simulink model "testingMotorModel"  (R2020b)
settings: Solver=VariableStepAuto  StartTime=0.0  StopTime=10  RelTol=1e-3
values from neighbouring files (symbols this model uses):
  A = motorSS.A    [doingActualControlTheory.m]
  B = motorSS.B    [doingActualControlTheory.m]
  C = motorSS.C    [doingActualControlTheory.m]
  D = motorSS.D    [doingActualControlTheory.m]
  Kr = K(1)    [doingActualControlTheory.m]
  Kx = K(2)    [doingActualControlTheory.m]
settings Model: Creator=drago  LastModifiedBy=drago

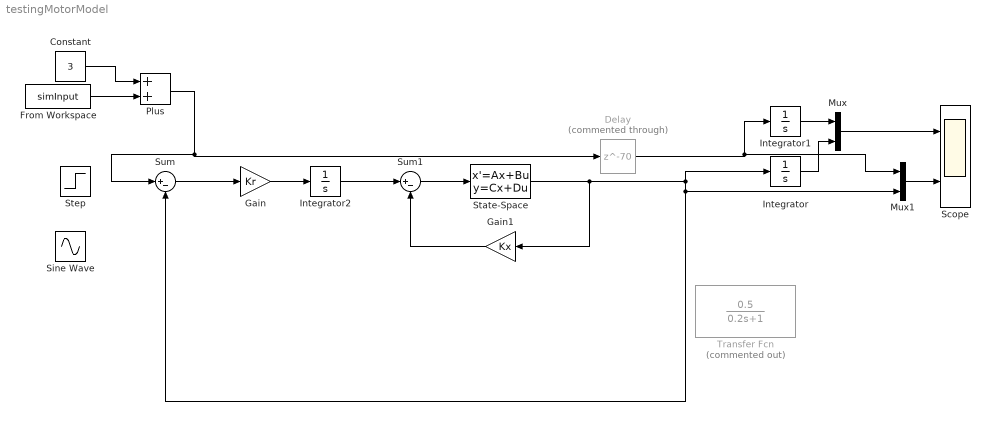
== system testingMotorModel ==
  Constant : Constant  Value=3
  Delay : Delay  Commented=through  DelayLength=70  SampleTime=0.01
  From Workspace : FromWorkspace  VariableName=simInput
  Gain : Gain  Gain=Kr
  Gain1 : Gain  Gain=Kx
  Integrator : Integrator
  Integrator1 : Integrator
  Integrator2 : Integrator
  Mux : Mux  Inputs=2
  Mux1 : Mux  Inputs=2
  Plus : Sum
  Scope : Scope  NumInputPorts=2
  Sine Wave : Sin  Frequency=0.1  SampleTime=0
  State-Space : StateSpace  A=A  B=B  C=C  D=D  InitialCondition=0
  Step : Step  Time=5  Before=10  SampleTime=0
  Sum : Sum  Inputs=|+-
  Sum1 : Sum  Inputs=|+-
  Transfer Fcn : TransferFcn  Commented=on  Numerator=[0.5]  Denominator=[0.2 1]
  wires:
  Plus/1 -> Sum/1, Delay/1
  Integrator/1 -> Mux/2
  Integrator1/1 -> Mux/1
  Mux/1 -> Scope/1
  Mux1/1 -> Scope/2
  Integrator2/1 -> Sum1/1
  Sum/1 -> Gain/1
  State-Space/1 -> Gain1/1, Mux1/2, Sum/2, Integrator/1
  Gain/1 -> Integrator2/1
  Gain1/1 -> Sum1/2
  Sum1/1 -> State-Space/1
  Constant/1 -> Plus/1
  From Workspace/1 -> Plus/2
  Delay/1 -> Integrator1/1, Mux1/1
